simulink model "Control_Selection_test"  (R2016b)
settings: Solver=VariableStepAuto  StartTime=0.0  StopTime=6400  RelTol=1e-3
libraries: control_selection x1
settings Model: Creator=Sean  LastModifiedBy=Sean

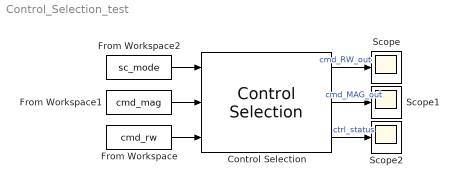
== system Control_Selection_test ==
  Control Selection : control_selection/control_selection/Control Selection
  From Workspace : FromWorkspace  VariableName=cmd_rw  SampleTime=0
  From Workspace1 : FromWorkspace  VariableName=cmd_mag  SampleTime=0
  From Workspace2 : FromWorkspace  VariableName=sc_mode  SampleTime=0
  Scope : Scope
  Scope1 : Scope
  Scope2 : Scope
  wires:
  From Workspace/1 -> Control Selection/3
  Control Selection/1 -> Scope/1  "cmd_RW_out"
  Control Selection/2 -> Scope1/1  "cmd_MAG_out"
  Control Selection/3 -> Scope2/1  "ctrl_status"
  From Workspace1/1 -> Control Selection/2
  From Workspace2/1 -> Control Selection/1
